simulink model "VFmodel"  (R2019a)
settings: Solver=VariableStepAuto  StartTime=0.0  StopTime=20  FixedStep=Simulation_step  MaxStep=Tc/2  RelTol=1e-3
values from neighbouring files (symbols this model uses):
  a = tau/(Ts_ctrl+tau)    (= 0.997493026589)    [VF_param.m]    (also in VF_param1.m = 0.987589583282)
  b = Ts_ctrl/(Ts_ctrl+tau)    (= 0.00250697341147)    [VF_param.m]    (also in VF_param1.m = 0.0124104167184)
  D = 1e-4    (= 0.0001)    [VF_param.m]    (also in VF_param1.m)
  J = 2e-4    (= 0.0002)    [VF_param.m]    (also in VF_param1.m)
  K_Idelta = 10    [VF_param.m]    (also in VF_param1.m)
  Ke = 0.8e-3    (= 0.0008)    [VF_param.m]    (also in VF_param1.m)
  Ld = L    (= 2e-05)    [VF_param.m]    (also in VF_param1.m)
  Lq = L    (= 2e-05)    [VF_param.m]    (also in VF_param1.m)
  Pn = 7    [VF_param.m]    (also in VF_param1.m)
  R = 20e-3    (= 0.02)    [VF_param.m]    (also in VF_param1.m)
  Tc = 1 / Fc    (= 0.001)    [VF_param1.m]
undefined symbols (not defined in the file or in its folder): DiscIntNeverNeededParam
settings Model: Creator=r720r  LastModifiedBy=r720r

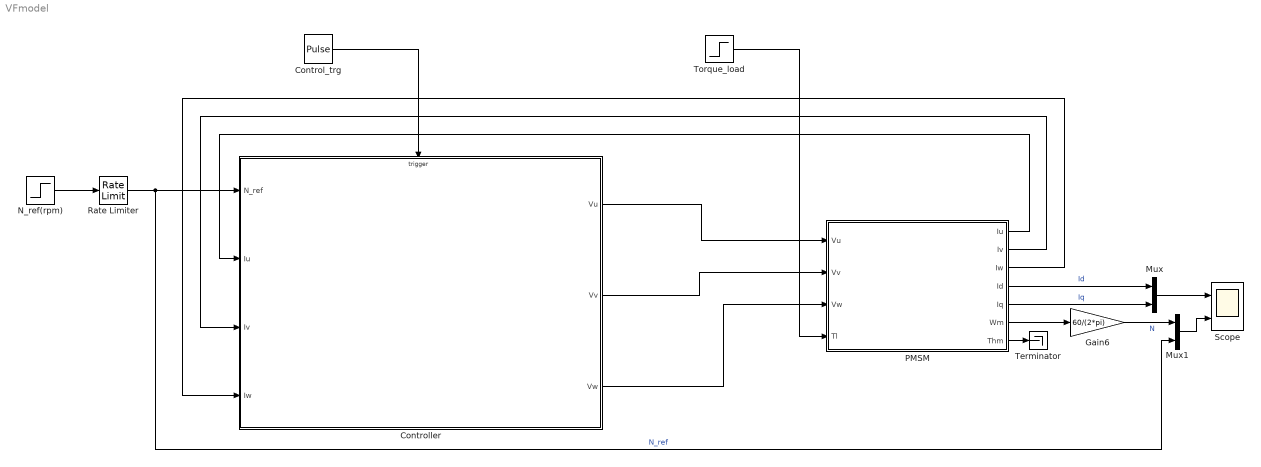
== system VFmodel ==
  Control_trg : DiscretePulseGenerator  PulseType=Time based  Period=Tc  PulseWidth=50
  Controller : Subsystem
  Gain6 : Gain  Gain=60/(2*pi)
  Mux : Mux  Inputs=2
  Mux1 : Mux  Inputs=2
  N_ref(rpm) : Step  Time=2  After=1000  SampleTime=0
  PMSM : Subsystem
  Rate Limiter : RateLimiter  RisingSlewLimit=200  FallingSlewLimit=-100  SampleTimeMode=inherited
  Scope : Scope  NumInputPorts=2
  Terminator : Terminator
  Torque_load : Step  Time=17  After=0.01  SampleTime=0
  wires:
  PMSM/6(Wm) -> Gain6/1
  PMSM/4(Id) -> Mux/1  "Id"
  PMSM/5(Iq) -> Mux/2  "Iq"
  Torque_load/1 -> PMSM/4(Tl)
  Gain6/1 -> Mux1/1  "N"
  PMSM/1(Iu) -> Controller/2(Iu)
  PMSM/2(Iv) -> Controller/3(Iv)
  PMSM/3(Iw) -> Controller/4(Iw)
  N_ref(rpm)/1 -> Rate Limiter/1
  Rate Limiter/1 -> Mux1/2, Controller/1(N_ref)  "N_ref"
  PMSM/7(Thm) -> Terminator/1
  Control_trg/1 -> Controller/Trigger
  Mux/1 -> Scope/1
  Mux1/1 -> Scope/2
  Controller/2(Vv) -> PMSM/2(Vv)
  Controller/1(Vu) -> PMSM/1(Vu)
  Controller/3(Vw) -> PMSM/3(Vw)

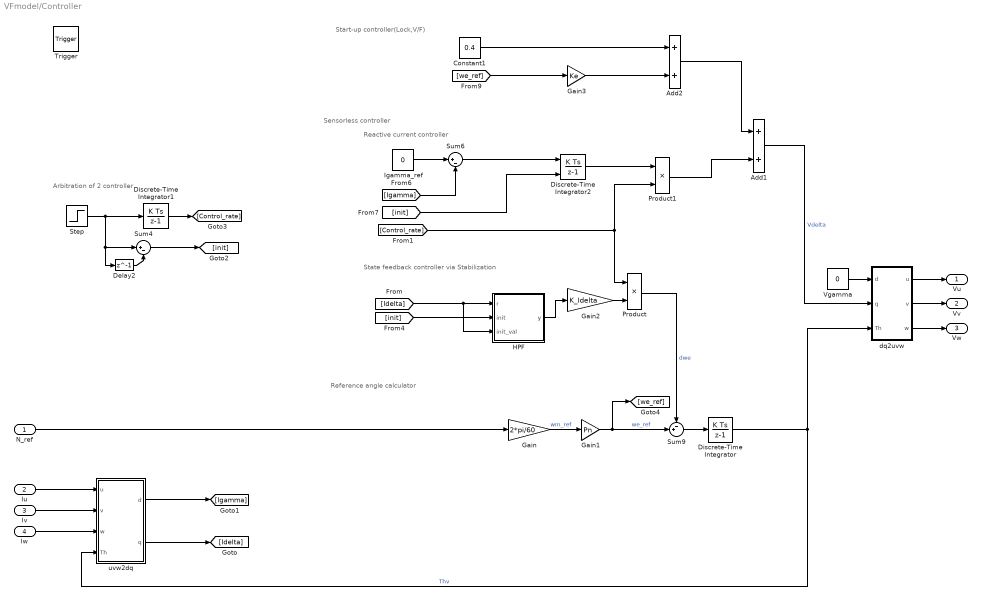
== system VFmodel/Controller ==
  note: Reference angle calculator
  note: Arbitration of 2 controller
  note: Sensorless controller
  note: Reactive current controller
  note: State feedback controller via Stabilization
  note: Start‐up controller(Lock,V/F)
  N_ref : Inport
  Iu : Inport  Port=2
  Iv : Inport  Port=3
  Iw : Inport  Port=4
  Trigger : TriggerPort  VariantControl=Variant  PortDimensions=1
  Add1 : Sum
  Add2 : Sum
  Constant1 : Constant  Value=0.4
  Delay2 : Delay  DelayLength=1
  Discrete-Time Integrator : DiscreteIntegrator  SampleTime=-1  ICPrevOutput=DiscIntNeverNeededParam  ICPrevScaledInput=DiscIntNeverNeededParam
  Discrete-Time Integrator1 : DiscreteIntegrator  gainval=0.5  SampleTime=-1  LimitOutput=on  UpperSaturationLimit=1  LowerSaturationLimit=-1  ICPrevOutput=DiscIntNeverNeededParam  ICPrevScaledInput=DiscIntNeverNeededParam
  Discrete-Time Integrator2 : DiscreteIntegrator  gainval=Ki_v  ExternalReset=rising  SampleTime=-1  ICPrevOutput=DiscIntNeverNeededParam  ICPrevScaledInput=DiscIntNeverNeededParam
  Gain : Gain  Gain=2*pi/60
  Gain1 : Gain  Gain=Pn
  Gain2 : Gain  Gain=K_Idelta
  Gain3 : Gain  Gain=Ke
  HPF : Subsystem
  Igamma_ref : Constant  Value=0
  Product : Product
  Product1 : Product
  Step : Step  Time=6
  Sum4 : Sum  Inputs=|+-
  Sum6 : Sum  Inputs=|+-
  Sum9 : Sum  Inputs=-+|
  Vgamma : Constant  Value=0
  dq2uvw : Subsystem
  uvw2dq : Subsystem
  Vu : Outport
  Vv : Outport  Port=2
  Vw : Outport  Port=3
  wires:
  Iu/1 -> uvw2dq/1(u)
  Sum9/1 -> Discrete-Time Integrator/1
  uvw2dq/1(d) -> [Igamma]
  Discrete-Time Integrator/1 -> uvw2dq/4(Th), dq2uvw/3(Th)  "Thv"
  Add2/1 -> Add1/1
  Product/1 -> Sum9/1  "dwe"
  Sum6/1 -> Discrete-Time Integrator2/1
  [Idelta] -> HPF/3(init_val), HPF/1(r)
  [Igamma] -> Sum6/2
  Iw/1 -> uvw2dq/3(w)
  Iv/1 -> uvw2dq/2(v)
  Gain1/1 -> Sum9/2, [we_ref]  "we_ref"
  N_ref/1 -> Gain/1
  Igamma_ref/1 -> Sum6/1
  HPF/1(y) -> Gain2/1
  Gain2/1 -> Product/2
  Gain/1 -> Gain1/1  "wm_ref"
  uvw2dq/2(q) -> [Idelta]
  Add1/1 -> dq2uvw/2(q)  "Vdelta"
  [init] -> HPF/2(init)
  Discrete-Time Integrator1/1 -> [Control_rate]
  Delay2/1 -> Sum4/2
  Sum4/1 -> [init]
  Step/1 -> Discrete-Time Integrator1/1, Delay2/1, Sum4/1
  [we_ref] -> Gain3/1
  Gain3/1 -> Add2/2
  Constant1/1 -> Add2/1
  Discrete-Time Integrator2/1 -> Product1/1
  [init] -> Discrete-Time Integrator2/2
  [Control_rate] -> Product/1, Product1/2
  Product1/1 -> Add1/2
  Vgamma/1 -> dq2uvw/1(d)
  dq2uvw/1(u) -> Vu/1
  dq2uvw/2(v) -> Vv/1
  dq2uvw/3(w) -> Vw/1

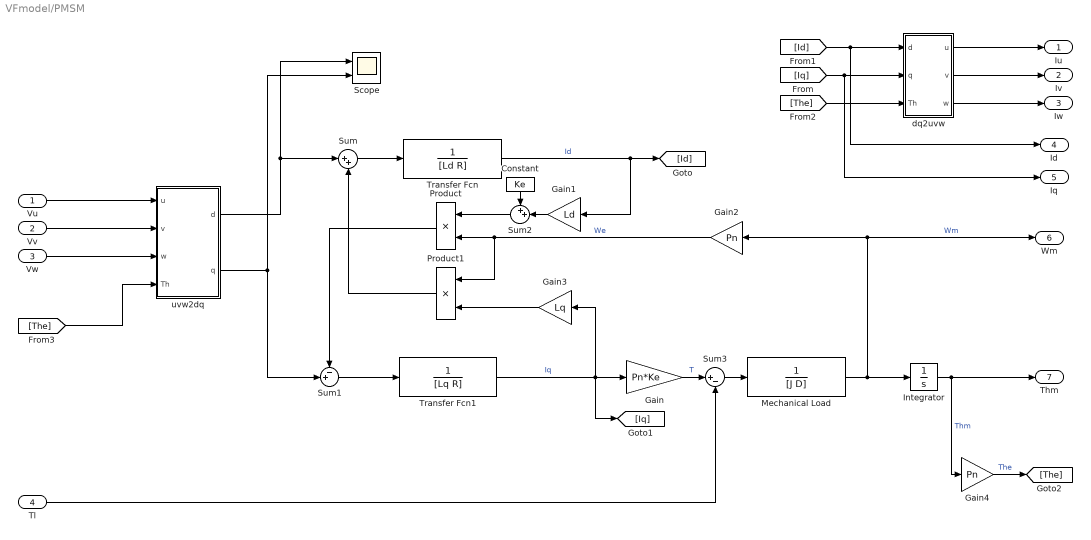
== system VFmodel/PMSM ==
  Vu : Inport
  Vv : Inport  Port=2
  Vw : Inport  Port=3
  Tl : Inport  Port=4
  Constant : Constant  Value=Ke
  Gain : Gain  Gain=Pn*Ke
  Gain1 : Gain  Gain=Ld
  Gain2 : Gain  Gain=Pn
  Gain3 : Gain  Gain=Lq
  Gain4 : Gain  Gain=Pn
  Integrator : Integrator
  Mechanical Load : TransferFcn  Denominator=[J D]
  Product : Product
  Product1 : Product
  Scope : Scope  NumInputPorts=2
  Sum : Sum  Inputs=|++
  Sum1 : Sum  Inputs=-+|
  Sum2 : Sum  Inputs=++|
  Sum3 : Sum  Inputs=|+-
  Transfer Fcn : TransferFcn  Denominator=[Ld R]
  Transfer Fcn1 : TransferFcn  Denominator=[Lq R]
  dq2uvw : Subsystem
  uvw2dq : Subsystem
  Iu : Outport
  Iv : Outport  Port=2
  Iw : Outport  Port=3
  Id : Outport  Port=4
  Iq : Outport  Port=5
  Wm : Outport  Port=6
  Thm : Outport  Port=7
  wires:
  Transfer Fcn1/1 -> Gain3/1, Gain/1, [Iq]  "Iq"
  Gain2/1 -> Product1/1, Product/2  "We"
  Gain1/1 -> Sum2/2
  Transfer Fcn/1 -> [Id], Gain1/1  "Id"
  Integrator/1 -> Thm/1, Gain4/1  "Thm"
  Gain/1 -> Sum3/1  "T"
  Sum/1 -> Transfer Fcn/1
  Sum2/1 -> Product/1
  [Iq] -> dq2uvw/2(q), Iq/1
  Mechanical Load/1 -> Integrator/1, Wm/1, Gain2/1  "Wm"
  Constant/1 -> Sum2/1
  Product1/1 -> Sum/2
  [Id] -> dq2uvw/1(d), Id/1
  Gain4/1 -> [The]  "The"
  Gain3/1 -> Product1/2
  Product/1 -> Sum1/1
  Sum1/1 -> Transfer Fcn1/1
  [The] -> dq2uvw/3(Th)
  dq2uvw/1(u) -> Iu/1
  dq2uvw/2(v) -> Iv/1
  dq2uvw/3(w) -> Iw/1
  Vu/1 -> uvw2dq/1(u)
  Vv/1 -> uvw2dq/2(v)
  Vw/1 -> uvw2dq/3(w)
  [The] -> uvw2dq/4(Th)
  uvw2dq/1(d) -> Scope/1, Sum/1
  uvw2dq/2(q) -> Scope/2, Sum1/2
  Sum3/1 -> Mechanical Load/1
  Tl/1 -> Sum3/2

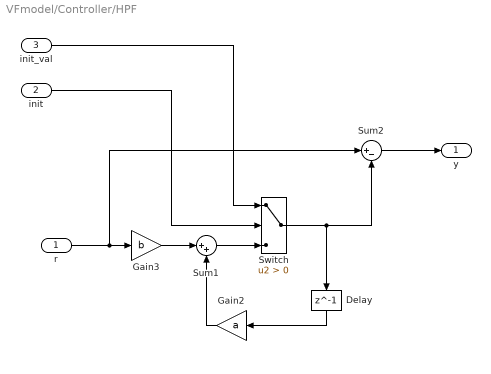
== system VFmodel/Controller/HPF ==
  r : Inport
  init : Inport  Port=2
  init_val : Inport  Port=3
  Delay : Delay  DelayLength=1
  Gain2 : Gain  Gain=a
  Gain3 : Gain  Gain=b
  Sum1 : Sum  Inputs=|++
  Sum2 : Sum  Inputs=|+-
  Switch : Switch  Criteria=u2 > Threshold
  y : Outport
  wires:
  Gain2/1 -> Sum1/2
  Sum2/1 -> y/1
  Sum1/1 -> Switch/3
  Switch/1 -> Sum2/2, Delay/1
  Gain3/1 -> Sum1/1
  r/1 -> Sum2/1, Gain3/1
  init_val/1 -> Switch/1
  Delay/1 -> Gain2/1
  init/1 -> Switch/2

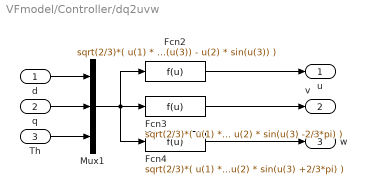
== system VFmodel/Controller/dq2uvw ==
  d : Inport
  q : Inport  Port=2
  Th : Inport  Port=3
  Fcn2 : Fcn  Expr=sqrt(2/3)*( u(1) * cos(u(3)) - u(2) * sin(u(3)) )
  Fcn3 : Fcn  Expr=sqrt(2/3)*( u(1) * cos(u(3)-2/3*pi) - u(2) * sin(u(3) -2/3*pi) )
  Fcn4 : Fcn  Expr=sqrt(2/3)*( u(1) * cos(u(3)+2/3*pi) - u(2) * sin(u(3) +2/3*pi) )
  Mux1 : Mux  Inputs=3
  u : Outport
  v : Outport  Port=2
  w : Outport  Port=3
  wires:
  d/1 -> Mux1/1
  Fcn4/1 -> w/1
  Fcn2/1 -> u/1
  Mux1/1 -> Fcn4/1, Fcn3/1, Fcn2/1
  q/1 -> Mux1/2
  Th/1 -> Mux1/3
  Fcn3/1 -> v/1

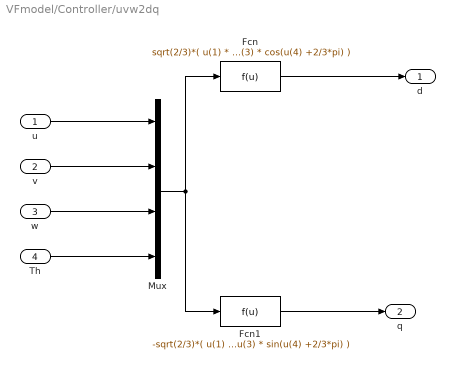
== system VFmodel/Controller/uvw2dq ==
  u : Inport
  v : Inport  Port=2
  w : Inport  Port=3
  Th : Inport  Port=4
  Fcn : Fcn  Expr=sqrt(2/3)*( u(1) * cos(u(4)) + u(2) * cos(u(4) - 2/3*pi) +u(3) * cos(u(4) +2/3*pi) )
  Fcn1 : Fcn  Expr=-sqrt(2/3)*( u(1) * sin(u(4)) + u(2) * sin(u(4) - 2/3*pi) +u(3) * sin(u(4) +2/3*pi) )
  Mux : Mux
  d : Outport
  q : Outport  Port=2
  wires:
  Fcn1/1 -> q/1
  w/1 -> Mux/3
  v/1 -> Mux/2
  Fcn/1 -> d/1
  Th/1 -> Mux/4
  Mux/1 -> Fcn1/1, Fcn/1
  u/1 -> Mux/1

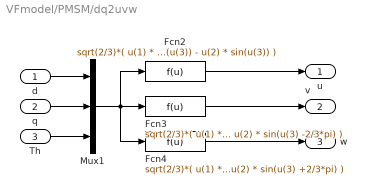
== system VFmodel/PMSM/dq2uvw ==
  d : Inport
  q : Inport  Port=2
  Th : Inport  Port=3
  Fcn2 : Fcn  Expr=sqrt(2/3)*( u(1) * cos(u(3)) - u(2) * sin(u(3)) )
  Fcn3 : Fcn  Expr=sqrt(2/3)*( u(1) * cos(u(3)-2/3*pi) - u(2) * sin(u(3) -2/3*pi) )
  Fcn4 : Fcn  Expr=sqrt(2/3)*( u(1) * cos(u(3)+2/3*pi) - u(2) * sin(u(3) +2/3*pi) )
  Mux1 : Mux  Inputs=3
  u : Outport
  v : Outport  Port=2
  w : Outport  Port=3
  wires:
  d/1 -> Mux1/1
  Fcn4/1 -> w/1
  Fcn2/1 -> u/1
  Mux1/1 -> Fcn4/1, Fcn3/1, Fcn2/1
  q/1 -> Mux1/2
  Th/1 -> Mux1/3
  Fcn3/1 -> v/1

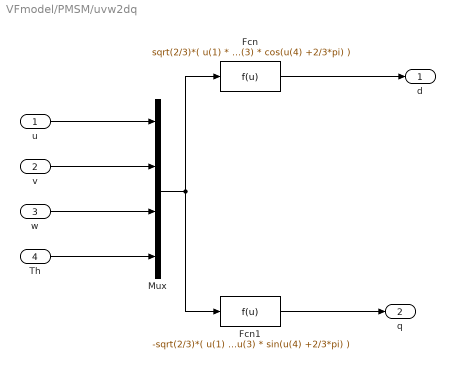
== system VFmodel/PMSM/uvw2dq ==
  u : Inport
  v : Inport  Port=2
  w : Inport  Port=3
  Th : Inport  Port=4
  Fcn : Fcn  Expr=sqrt(2/3)*( u(1) * cos(u(4)) + u(2) * cos(u(4) - 2/3*pi) +u(3) * cos(u(4) +2/3*pi) )
  Fcn1 : Fcn  Expr=-sqrt(2/3)*( u(1) * sin(u(4)) + u(2) * sin(u(4) - 2/3*pi) +u(3) * sin(u(4) +2/3*pi) )
  Mux : Mux
  d : Outport
  q : Outport  Port=2
  wires:
  Fcn1/1 -> q/1
  w/1 -> Mux/3
  v/1 -> Mux/2
  Fcn/1 -> d/1
  Th/1 -> Mux/4
  Mux/1 -> Fcn1/1, Fcn/1
  u/1 -> Mux/1
